simulink model "robot_aparalel"  (R2020b)
settings: Solver=VariableStepAuto  StartTime=0.0  StopTime=inf  RelTol=1e-3
libraries: simulink x4
settings Model: Creator=mihai  LastModifiedBy=mihai

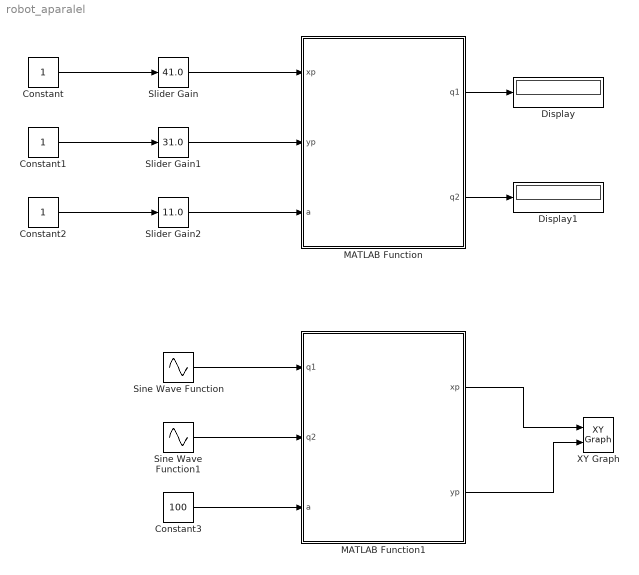
== system robot_aparalel ==
  Constant : Constant
  Constant1 : Constant
  Constant2 : Constant
  Constant3 : Constant  Value=100
  Display : Display
  Display1 : Display
  MATLAB Function : MATLAB Function  TreatAsAtomicUnit=on
  MATLAB Function1 : MATLAB Function  TreatAsAtomicUnit=on
  Sine Wave Function : Sin  Amplitude=10  SampleTime=0
  Sine Wave Function1 : Sin  Amplitude=10  Phase=pi/2  SampleTime=0
  Slider Gain : simulink/Math Operations/Slider Gain  gain=41.0  low=0  high=100
  Slider Gain1 : simulink/Math Operations/Slider Gain  gain=31.0  low=0  high=100
  Slider Gain2 : simulink/Math Operations/Slider Gain  gain=11.0  low=0  high=100
  XY Graph : simulink/Sinks/XY Graph  xmin=0  xmax=100  ymin=0  ymax=100  st=-1
  wires:
  MATLAB Function/1(q1) -> Display/1
  MATLAB Function/2(q2) -> Display1/1
  Constant/1 -> Slider Gain/1
  Constant1/1 -> Slider Gain1/1
  Constant2/1 -> Slider Gain2/1
  Slider Gain2/1 -> MATLAB Function/3(a)
  Slider Gain1/1 -> MATLAB Function/2(yp)
  Slider Gain/1 -> MATLAB Function/1(xp)
  MATLAB Function1/1(xp) -> XY Graph/1
  MATLAB Function1/2(yp) -> XY Graph/2
  Constant3/1 -> MATLAB Function1/3(a)
  Sine Wave Function/1 -> MATLAB Function1/1(q1)
  Sine Wave Function1/1 -> MATLAB Function1/2(q2)

== matlab function robot_aparalel/MATLAB Function1 ==
  data: q1 input; xp output; q2 input; a input; yp output
function [xp,yp] = fcn(q1,q2,a)

    xp = (q2^2-q1^2 - a^2)/(-2*a);
    yp = sqrt(abs(q1^2 -xp^2));

== matlab function robot_aparalel/MATLAB Function ==
  data: xp input; q1 output; yp input; a input; q2 output
function [q1,q2] = fcn(xp,yp,a)
    q1 = sqrt(xp^2 + yp^2);
    q2 = sqrt((a - xp)^2 + yp^2);
